simulink model "steering_pad_test_dual"  (R2024b)
settings: Solver=VariableStepAuto  StartTime=0.0  StopTime=10  FixedStep=0.001  RelTol=1e-4
undefined symbols (not defined in the file or in its folder): car
libraries: slpidlib x2, vehdynlibsteering x1, autolibshared x1
settings Model: Creator=Carlo  LastModifiedBy=Carlo
settings SolverCC: ZeroCrossAlgorithm=Adaptive
settings DebuggingCC: IgnoredZcDiagnostic=none

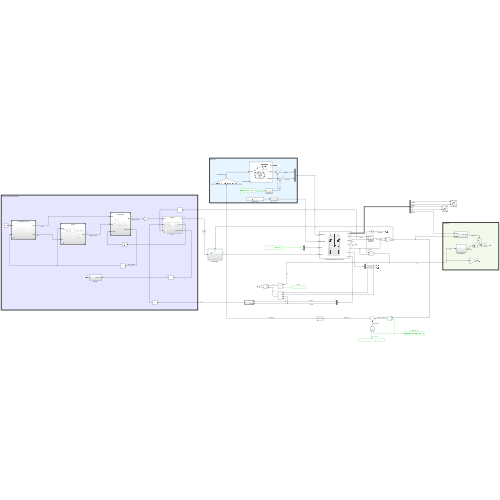
[thumbnail: Simulink's stored preview of the top-level diagram]
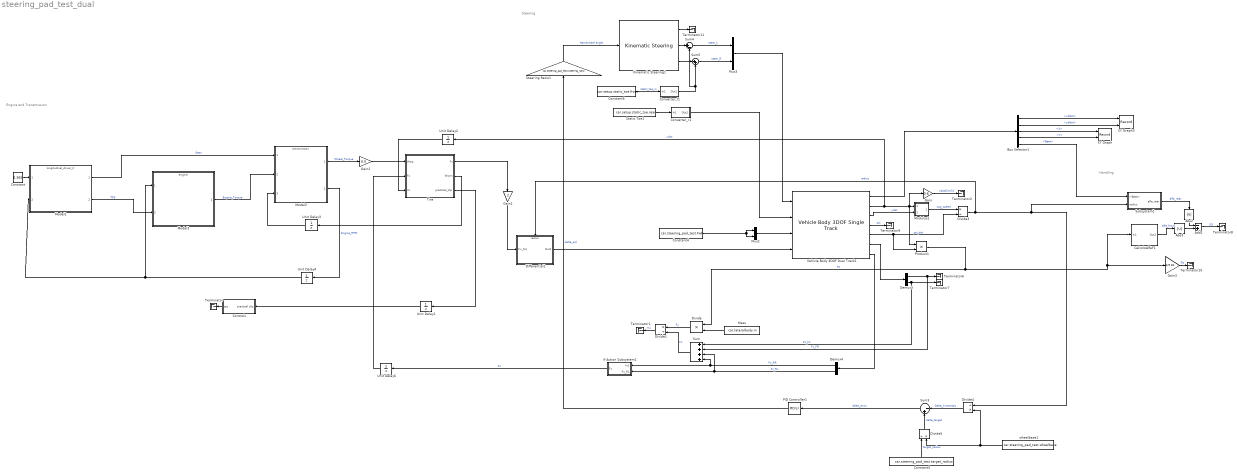
== system steering_pad_test_dual ==
  note: Handling
  note: Steering
  note: Engine and Transmission
  Abs2 : Abs  SaturateOnIntegerOverflow=off
  Abs3 : Abs  SaturateOnIntegerOverflow=off
  Add1 : Sum  Inputs=-+
  Bus Selector1 : BusSelector  OutputSignals=BdyFrm.Cg.Acc.xddot,BdyFrm.Cg.Acc.yddot,InertFrm.Cg.Disp.X,InertFrm.Cg.Disp.Y,BdyFrm.Geom.Ang.Beta
  CalcoloAlfaF1 : Subsystem
  Constant : Constant  Value=0.365
  Constant4 : Constant  Value=car.steering_pad_test.FwF
  Constant5 : Constant  Value=car.steering_pad_test.target_radius
  Constant6 : Constant  Value=car.setup.static_toe.front
  Controls : Subsystem
  Converter_f1 : Subsystem
  Converter_r1 : Subsystem
  Demux3 : Demux  Outputs=2
  Demux4 : Demux  Outputs=2
  Differential1 : Subsystem
      settings: PortSchema="{\"entries\":[{\"content\":{\"sides\":[{\"content\":{\"connectorIds\":[\"In1\"]},\"type\":\"ConnectorPlacement.EquallySpacedRectSide\",\"uuid\":\"e0135ed7-8abf-48dc-a26a-f2473ebc5583\"},{\"content\":{\"connectorIds\":[\"Out1\"],\"side\":\"RIGHT\"},\"type\":\"ConnectorPlacement.EquallySpacedRectSide\",\"uuid\":\"62eb6c38-b859-47c0-94be-9d58d81aad83\"},{\"content\":{\"connectorIds\":[\"In2\"],\"side\":\"TOP\"},\"type\":\"ConnectorPlacement.EquallySpacedRectSide\",\"uuid\":\"7d57c051-97d0-4363-afda-d558cd95b86e\"},{\"content\":{\"side\":\"BOTTOM\"},\"type\":\"ConnectorPlacement.EquallySpacedRectSide\",\"uuid\":\"2453ae4c-76f8-40d8-a1dc-17514a77823a\"}]},\"type\":\"ConnectorPlacement.EquallySpacedConnector\",\"uuid\":\"6460a95d-0a38-4080-9ca3-bbd140d34657\"}],\"packageUris\":[\"http://schema.mathworks.com/mf0/Connector/R2020b\"],\"version\":\"1.0\"}"
  Divide : Product  Inputs=**
  Divide1 : Product  Inputs=*/
  Divide3 : Product  Inputs=*/
  Divide4 : Product  Inputs=/*
  Divide5 : Product  Inputs=/*
  Gain : Gain  Gain=3.6
  Gain1 : Gain  Gain=2
  Gain2 : Gain  Gain=0.5
  Gain3 : Gain  Gain=1/9.81
  If Action Subsystem1 : Subsystem  TreatAsAtomicUnit=on
  Kinematic Steering1 : vehdynlibsteering/Kinematic Steering  StrgType=Ackerman  StrgRatioType=Constant  Loc=Front  NrmlFctr=car.kinematic_steering.NrmlFctr  TrckWdth=car.kinematic_steering.TrckWdth  WhlBase=car.kinematic_steering.WhlBase  Db=car.kinematic_steering.Db  StrgRng=car.kinematic_steering.StrgRng  StrgAngBpts="[-6.2832   -5.0265   -3.7699   -2.5133   -1.2566         0    1.2566    2.5133    3.7699    5.0265    6.2832]"  StrgRatioTbl=|  StrgRatio=car.kinematic_steering.StrgRatio  PctAckIn=off  PctAck=car.kinematic_steering.PctAck  PctAckTbl=ones(1,11)*100  StrgArmLngth=0.1  RckCsLngth=0.5  TieRodLngth=0.248  D=0.2  PnnRadius=0.00085818  PnnRadiusTbl="[0.0055    0.0055    0.0056    0.0057    0.0058    0.0057    0.0057    0.0057    0.0056    0.0055    0.0055]"  RodLngth=0.1  ParaArmLngth=0.9  aMode=2
      | [13.5000   13.3750   13.2500   13.1250   13.0000   13.0000   13.0000   13.1250   13.2500   13.3750   13.5000
      | ]
  Mass : Constant  Value=car.lateralbody.m
  Model1 : ModelReference  ModelNameDialog=longitudinal_driver_2.slx  SimulationMode=Normal  ModelReferenceVersion=1.7
  Model2 : ModelReference  ModelNameDialog=transmission.slx  SimulationMode=Normal  ModelReferenceVersion=1.12
  Model3 : ModelReference  ModelNameDialog=engine.slx  SimulationMode=Normal  ModelReferenceVersion=1.18
  Modulus1 : Subsystem
  Mux2 : Mux  Inputs=2
  Mux3 : Mux  Inputs=2
  PID Controller1 : slpidlib/PID Controller  Controller=PID  Form=Parallel  TimeDomain=Continuous-time  UseExternalTs=off  SampleTime=-1  IntegratorMethod=Forward Euler  FilterMethod=Forward Euler  ControllerParametersSource=internal  P=car.steering_pad_test.PID.P  I=car.steering_pad_test.PID.I  UseKiTs=off  D=car.steering_pad_test.PID.D  UseExternalDerivativeSource=off  N=car.steering_pad_test.PID.N  UseFilter=on  TunerSelectOption=Transfer Function Based (PID Tuner App)  InitialConditionSource=internal  InitialConditionForIntegrator=0  InitialConditionForFilter=0  DifferentiatorICPrevScaledInput=0  ExternalReset=none  TrackingMode=off  Kt=1  LimitOutput=off  SatLimitsSource=internal  UpperSaturationLimit=inf  LowerSaturationLimit=-inf  LinearizeAsGain=on  AntiWindupMode=none  Kb=1  LimitIntegrator=off  UpperIntegratorSaturationLimit=inf  LowerIntegratorSaturationLimit=-inf  POutMin=[]  POutMax=[]  IOutMin=[]  IOutMax=[]  DOutMin=[]  DOutMax=[]  NOutMin=[]  NOutMax=[]  SumOutMin=[]  SumOutMax=[]  SaturationOutMin=[]  SaturationOutMax=[]  PParamMin=[]  PParamMax=[]  IParamMin=[]  IParamMax=[]  DParamMin=[]  DParamMax=[]  NParamMin=[]  NParamMax=[]  KbParamMin=[]  KbParamMax=[]  KtParamMin=[]  KtParamMax=[]  KbOutMin=[]  KbOutMax=[]  KtOutMin=[]  KtOutMax=[]  IntegratorOutMin=[]  IntegratorOutMax=[]  FilterOutMin=[]  FilterOutMax=[]  SumI1OutMin=[]  SumI1OutMax=[]  SumI2OutMin=[]  SumI2OutMax=[]  SumI3OutMin=[]  SumI3OutMax=[]  SumI4OutMin=[]  SumI4OutMax=[]  SumDOutMin=[]  SumDOutMax=[]  DifferentiatorOutMin=[]  DifferentiatorOutMax=[]  FilterDiffOutCoefMin=[]  FilterDiffOutCoefMax=[]  ReciprocalOutMin=[]  ReciprocalOutMax=[]  SumDenOutMin=[]  SumDenOutMax=[]  SumNumOutMin=[]  SumNumOutMax=[]  DivideOutMin=[]  DivideOutMax=[]  UdiffTsProdOutMin=[]  UdiffTsProdOutMax=[]  NTsProdOutMin=[]  NTsProdOutMax=[]  UintegralTsProdOutMin=[]  UintegralTsProdOutMax=[]  UngainTsProdOutMin=[]  UngainTsProdOutMax=[]  ClampingZeroOutDataTypeStr=Inherit: Inherit via back propagation  ClampingZeroOutMin=[]  ClampingZeroOutMax=[]  FilterDenConstantOutDataTypeStr=Inherit: Inherit via back propagation  FilterDenConstantOutMin=[]  FilterDenConstantOutMax=[]  PCopyOutDataTypeStr=Inherit: Inherit via back propagation  PCopyOutMin=[]  PCopyOutMax=[]  NCopyOutDataTypeStr=Inherit: Inherit via back propagation  NCopyOutMin=[]  NCopyOutMax=[]  IntegratorContinuousStateAttributes=''  IntegratorStateMustResolveToSignalObject=off  IntegratorRTWStateStorageClass=Auto  FilterContinuousStateAttributes=''  FilterStateMustResolveToSignalObject=off  FilterRTWStateStorageClass=Auto  ParallelPVariant=InternalParameters  IdealPVariant=Disabled  IVariant=InternalParameters  DVariant=InternalParameters  IntegratorVariant=Continuous  SatVariant=Disabled  AWVariant=Passthrough  PCopyVariant=Disabled  TRVariant=Disabled  FdbkBlocksVariant=Forward  IdealPFdbkVariant=Disabled  SatFdbkVariant=Disabled  DerivativeFilterVariant=ContFilter  NVariant=InternalParameters  NCopyVariant=Disabled  FilterICVariant=InternalICsFilter  IntegratorICVariant=InternalICs  ExternalResetVariant=Disabled  TRSumVariant=Passthrough  SumFdbkVariant=Disabled  SumVariant=Sum_PID  TsampFilterVariant=InternalTs  TsampNgainVariant=Passthrough  TsampIntegralVariant=Disabled_SignalSpec  ExternalSaturationOutDataTypeStr=Inherit: Same as second input  DerivativeSourceVariant=ErrorSignal  PreIntVariant=InternalPreInt
  Product1 : Product
  Static Toe1 : Constant  Value=car.setup.static_toe.rear
  Steering Ratio1 : Gain  Gain=car.steering_pad_test.steering_ratio
  Subsystem1 : Subsystem
  Sum : Sum  Inputs=++++
  Sum3 : Sum  Inputs=|-+
  Sum4 : Sum  Inputs=|+-
  Sum5 : Sum  Inputs=|++
  Terminator{,1..2,6..11} (9 alike) : Terminator
  Tire : Subsystem  Variant=on
  Unit Delay1 : UnitDelay  SampleTime=-1  HasFrameUpgradeWarning=on
  Unit Delay2 : UnitDelay  InitialCondition=car.initialconditions.xdot  SampleTime=-1  HasFrameUpgradeWarning=on
  Unit Delay3 : UnitDelay  InitialCondition=car.initialconditions.Wrpm  SampleTime=-1  HasFrameUpgradeWarning=on
  Unit Delay4 : UnitDelay  InitialCondition=car.initialconditions.EngineRPM  SampleTime=-1  HasFrameUpgradeWarning=on
  Unit Delay6 : UnitDelay  SampleTime=-1  HasFrameUpgradeWarning=on
  Vehicle Body 3DOF Dual Track1 : autolibshared/Vehicle Body 3DOF Single Track  trackMode=Dual  inputMode=External longitudinal forces  frontSteerMode=on  rearSteerMode=on  windMode=off  muMode=off  extFMode=off  extMMode=off  htchFMode=off  htchMMode=off  extXo=off  extpsio=off  extxdoto=off  extro=off  extYo=off  extTamb=off  extydoto=off  aMode=2  NF=car.lateralbody.NF  NR=car.lateralbody.NR  m=car.lateralbody.m  a=car.lateralbody.a  b=car.lateralbody.b  h=car.lateralbody.h  dh=1  hh=0.2  X_o=car.lateralbody.X_o  xdot_o=car.lateralbody.xdot_o  CalphaMode=off  sigmaMode=on  d=car.lateralbody.d  hl=0  w=car.lateral.body.w  Cy_f=car.lateralbody.Cy_f  Cy_r=car.lateralbody.Cy_r  sigma_f=car.lateralbody.sigma_f  sigma_r=car.lateralbody.sigma_r  alpha_f_brk=[-.1 .1]  Cy_f_data=[-9e3 9e3]  alpha_r_brk=[-.1 .1]  Cy_r_data=[-9e3 9e3]  Y_o=car.lateralbody.Y_o  ydot_o=car.lateralbody.ydot_o  Izz=car.lateralbody.Izz  psi_o=car.lateralbody.psi_o  r_o=car.lateralbody.r_o  Af=car.lateralbody.Af  Cd=car.lateralbody.Cd  Cl=car.lateralbody.Cl  Cpm=car.lateralbody.Cpm  beta_w=car.lateralbody.beta_w  Cs=car.lateralbody.Cs  Cym=car.lateralbody.Cym  Pabs=car.lateralbody.Pabs  Tair=car.lateralbody.Tair  g=car.lateralbody.g  mu=car.lateralbody.mu  xdot_tol=car.lateralbody.xdot_tol  Fznom=car.lateralbody.Fznom  Fxtire_sat=7e4  Fytire_sat=7e4  longOff=car.lateralbody.longOff  latOff=car.lateralbody.latOff  vertOff=car.lateralbody.vertOff  wrapAng=off
      settings: LibrarySourceBlock=vehdynlibeom/Vehicle Body 3DOF Dual Track
  XY Graph : Record  FileSettingsInternal="{\"entries\":[{\"content\":{\"excelSettings\":{\"content\":{},\"type\":\"Streamout.ExcelSettings\"}},\"type\":\"Streamout.FileSettingStorage\",\"uuid\":\"\"}],\"packageUris\":[\"http:\\/\\/schema.mathworks.com\\/mf0\\/streamout_blocks\\/R2020a\"],\"version\":\"1.0\"}"  Layout=[1 1]  SignalsInternal="{\"entries\":[{\"content\":{\"signals\":[{\"content\":{\"blockPath\":[],\"dimensions\":[1],\"domain\":\"\",\"lineColor\":\"#a2142f\",\"plots\":[ 1 ],\"port\":1,\"sid\":[\"\"],\"signalID\":1,\"signalName\":\"<X>\"},\"type\":\"RecordBlkView.Signal\",\"uuid\":\"\"},{\"content\":{\"blockPath\":[],\"dimensions\":[1],\"domain\":\"\",\"lineColor\":\"#139fff\",\"plots\":[ 1 ],\"port\":2,\"sid\":[\"\"],\"signalID\":2,\"signalName\":\"<Y>\"},\"type\":\"RecordBlkView.Signal\",\"uuid\":\"\"}]},\"type\":\"RecordBlkView.InputSignals\",\"uuid\":\"\"}],\"packageUris\":[\"http:\\/\\/schema.mathworks.com\\/mf0\\/streamout_blocks\\/R2020a\"],\"version\":\"1.0\"}"  VisualizationBindings="{\"xyplotplugin\":{\"info\":[{\"series\":[{\"bindingParametersList\":[{\"parameter\":\"X-Axis\",\"signalID\":1,\"signalName\":\"<X>\"},{\"parameter\":\"Y-Axis\",\"signalID\":2,\"signalName\":\"<Y>\"}],\"seriesID\":0}],\"subplotID\":1}]}}"  CompatibilityTag=XY
  XY Graph3 : Record  FileSettingsInternal="{\"entries\":[{\"content\":{\"excelSettings\":{\"content\":{},\"type\":\"Streamout.ExcelSettings\"}},\"type\":\"Streamout.FileSettingStorage\",\"uuid\":\"\"}],\"packageUris\":[\"http:\\/\\/schema.mathworks.com\\/mf0\\/streamout_blocks\\/R2020a\"],\"version\":\"1.0\"}"  Layout=[1 1]  SignalsInternal="{\"entries\":[{\"content\":{\"signals\":[{\"content\":{\"blockPath\":[],\"dimensions\":[1],\"domain\":\"\",\"lineColor\":\"#fe330a\",\"lineWidth\":2,\"port\":1,\"sid\":[\"\"],\"signalID\":1,\"signalName\":\"<xddot>\"},\"type\":\"RecordBlkView.Signal\",\"uuid\":\"\"},{\"content\":{\"blockPath\":[],\"dimensions\":[1],\"domain\":\"\",\"lineColor\":\"#22b573\",\"lineWidth\":2,\"port\":2,\"sid\":[\"\"],\"signalID\":2,\"signalName\":\"<yddot>\"},\"type\":\"RecordBlkView.Signal\",\"uuid\":\"\"}]},\"type\":\"RecordBlkView.InputSignals\",\"uuid\":\"\"}],\"packageUris\":[\"http:\\/\\/schema.mathworks.com\\/mf0\\/streamout_blocks\\/R2020a\"],\"version\":\"1.0\"}"  VisualizationBindings="{\"xyplotplugin\":{\"info\":[{\"series\":[],\"subplotID\":1}]}}"  CompatibilityTag=XY
  wheelbase1 : Constant  Value=car.steering_pad_test.wheelbase
  wires:
  Unit Delay3/1 -> Model2/3
  Model1/2 -> Model3/2  "TPS"
  Unit Delay4/1 -> Model3/1, Model1/2
  Unit Delay1/1 -> Controls/1(practical slip)
  Tire/3(practical_slip) -> Unit Delay1/1
  Model3/1 -> Model2/2  "Engine_Torque"
  Unit Delay2/1 -> Tire/3(Vx)
  Model1/1 -> Model2/1  "Gear"
  Tire/2(Wrpm) -> Unit Delay3/1
  Model2/1 -> Gain2/1  "Wheel_Torque"
  Model2/2 -> Unit Delay4/1  "Engine_RPM"
  Gain2/1 -> Tire/1(Wtrq)
  Sum3/1 -> PID Controller1/1  "delta_error"
  Bus Selector1/1 -> XY Graph3/1  "<xddot>"
  Modulus1/1(Out1) -> Divide3/1  "cog_speed"
  Bus Selector1/4 -> XY Graph/2  "<Y>"
  PID Controller1/1 -> Steering Ratio1/1  "delta_pid"
  Vehicle Body 3DOF Dual Track1/6 -> Demux3/1
  Bus Selector1/5 -> Subsystem1/1(<Beta>)  "<Beta>"
  Kinematic Steering1/1 -> Terminator11/1
  Bus Selector1/2 -> XY Graph3/2  "<yddot>"
  Divide5/1 -> Sum3/2  "delta_target"
  CalcoloAlfaF1/1(Out1) -> Abs3/1  "alfa_front"
  Constant4/1 -> Mux2/2, Mux2/1
  Constant5/1 -> Divide5/1  "target_radius"
  Subsystem1/1(alfa_rear) -> Abs2/1  "alfa_rear"
  Divide4/1 -> Sum3/1  "Delta_kinematic"
  Mux3/1 -> Vehicle Body 3DOF Dual Track1/1
  Vehicle Body 3DOF Dual Track1/1 -> Bus Selector1/1
  Abs3/1 -> Add1/2
  Sum5/1 -> Mux3/2  "steer_R"
  Kinematic Steering1/3 -> Sum5/1
  Divide3/1 -> Subsystem1/2(radius), Divide4/1, Differential1/2(radius)  "radius"
  Vehicle Body 3DOF Dual Track1/4 -> Terminator9/1  "psi"
  Mux2/1 -> Vehicle Body 3DOF Dual Track1/3
  Vehicle Body 3DOF Dual Track1/2 -> Unit Delay2/1, Gain/1, Modulus1/1(<xdot>), Product1/1  "xdot"
  Differential1/1(Out1) -> Vehicle Body 3DOF Dual Track1/4
  Add1/1 -> Terminator8/1  "US"
  Demux3/1 -> Sum/2, Terminator6/1  "Fz_FR"
  wheelbase1/1 -> Divide4/2, Divide5/2
  Demux3/2 -> Sum/1, Terminator7/1  "Fz_FL"
  Sum4/1 -> Mux3/1  "steer_L"
  Converter_f1/1(Out1) -> Sum4/2, Sum5/2
  Vehicle Body 3DOF Dual Track1/5 -> Product1/2, Divide3/2  "psi_dot"
  Static Toe1/1 -> Converter_r1/1(In1)
  Constant6/1 -> Converter_f1/1(In1)  "static_toe_in"
  Bus Selector1/3 -> XY Graph/1  "<X>"
  Converter_r1/1(Out1) -> Vehicle Body 3DOF Dual Track1/2
  Product1/1 -> Divide/1, CalcoloAlfaF1/1(In1), Gain3/1  "ay"
  Vehicle Body 3DOF Dual Track1/3 -> Modulus1/2(<ydot>)  "ydot"
  Gain3/1 -> Terminator10/1  "Gy"
  Abs2/1 -> Add1/1
  Steering Ratio1/1 -> Kinematic Steering1/1  "Handwheel angle"
  Kinematic Steering1/2 -> Sum4/1
  Demux4/1 -> Sum/4, If Action Subsystem1/1(In1)  "Fz_RR"
  Vehicle Body 3DOF Dual Track1/7 -> Demux4/1
  Demux4/2 -> Sum/3, If Action Subsystem1/2(Fz_RL)  "Fz_RL"
  If Action Subsystem1/1(Fz) -> Unit Delay6/1  "Fz"
  Unit Delay6/1 -> Tire/2(Fz)
  Constant/1 -> Model1/1
  Tire/1(Fx) -> Gain1/1
  Gain1/1 -> Differential1/1(Fx_tot)
  Controls/1(tps) -> Terminator/1
  Mass/1 -> Divide/2
  Divide/1 -> Divide1/1  "Fy"
  Divide1/1 -> Terminator1/1  "mu"
  Gain/1 -> Terminator2/1  "xdot[km/h]"
  Sum/1 -> Divide1/2  "Fz"

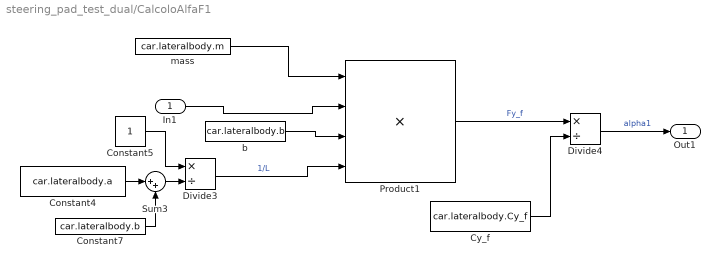
== system steering_pad_test_dual/CalcoloAlfaF1 ==
  In1 : Inport
  Constant4 : Constant  Value=car.lateralbody.a
  Constant5 : Constant
  Constant7 : Constant  Value=car.lateralbody.b
  Cy_f : Constant  Value=car.lateralbody.Cy_f
  Divide3 : Product  Inputs=*/
  Divide4 : Product  Inputs=*/
  Product1 : Product  Inputs=4
  Sum3 : Sum  Inputs=|++
  b : Constant  Value=car.lateralbody.b
  mass : Constant  Value=car.lateralbody.m
  Out1 : Outport
  wires:
  mass/1 -> Product1/1
  Divide3/1 -> Product1/4  "1/L"
  Sum3/1 -> Divide3/2
  b/1 -> Product1/3
  Constant4/1 -> Sum3/1
  Constant5/1 -> Divide3/1
  Divide4/1 -> Out1/1  "alpha1"
  Constant7/1 -> Sum3/2
  Product1/1 -> Divide4/1  "Fy_f"
  Cy_f/1 -> Divide4/2
  In1/1 -> Product1/2

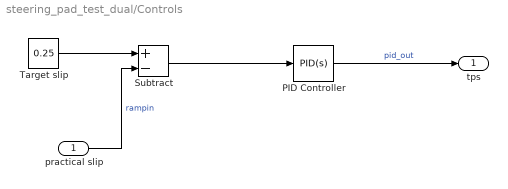
== system steering_pad_test_dual/Controls ==
  practical slip : Inport
  PID Controller : slpidlib/PID Controller  Controller=PID  Form=Parallel  TimeDomain=Continuous-time  UseExternalTs=off  SampleTime=-1  IntegratorMethod=Forward Euler  FilterMethod=Forward Euler  ControllerParametersSource=internal  P=7.5  I=0.75  UseKiTs=off  D=0.075  UseExternalDerivativeSource=off  N=0  UseFilter=on  TunerSelectOption=Transfer Function Based (PID Tuner App)  InitialConditionSource=internal  InitialConditionForIntegrator=0  InitialConditionForFilter=0  DifferentiatorICPrevScaledInput=0  ExternalReset=none  TrackingMode=off  Kt=1  LimitOutput=on  SatLimitsSource=internal  UpperSaturationLimit=1  LowerSaturationLimit=0  LinearizeAsGain=on  AntiWindupMode=none  Kb=1  LimitIntegrator=off  UpperIntegratorSaturationLimit=inf  LowerIntegratorSaturationLimit=-inf  POutMin=[]  POutMax=[]  IOutMin=[]  IOutMax=[]  DOutMin=[]  DOutMax=[]  NOutMin=[]  NOutMax=[]  SumOutMin=[]  SumOutMax=[]  SaturationOutMin=[]  SaturationOutMax=[]  PParamMin=[]  PParamMax=[]  IParamMin=[]  IParamMax=[]  DParamMin=[]  DParamMax=[]  NParamMin=[]  NParamMax=[]  KbParamMin=[]  KbParamMax=[]  KtParamMin=[]  KtParamMax=[]  KbOutMin=[]  KbOutMax=[]  KtOutMin=[]  KtOutMax=[]  IntegratorOutMin=[]  IntegratorOutMax=[]  FilterOutMin=[]  FilterOutMax=[]  SumI1OutMin=[]  SumI1OutMax=[]  SumI2OutMin=[]  SumI2OutMax=[]  SumI3OutMin=[]  SumI3OutMax=[]  SumI4OutMin=[]  SumI4OutMax=[]  SumDOutMin=[]  SumDOutMax=[]  DifferentiatorOutMin=[]  DifferentiatorOutMax=[]  FilterDiffOutCoefMin=[]  FilterDiffOutCoefMax=[]  ReciprocalOutMin=[]  ReciprocalOutMax=[]  SumDenOutMin=[]  SumDenOutMax=[]  SumNumOutMin=[]  SumNumOutMax=[]  DivideOutMin=[]  DivideOutMax=[]  UdiffTsProdOutMin=[]  UdiffTsProdOutMax=[]  NTsProdOutMin=[]  NTsProdOutMax=[]  UintegralTsProdOutMin=[]  UintegralTsProdOutMax=[]  UngainTsProdOutMin=[]  UngainTsProdOutMax=[]  ClampingZeroOutDataTypeStr=Inherit: Inherit via back propagation  ClampingZeroOutMin=[]  ClampingZeroOutMax=[]  FilterDenConstantOutDataTypeStr=Inherit: Inherit via back propagation  FilterDenConstantOutMin=[]  FilterDenConstantOutMax=[]  PCopyOutDataTypeStr=Inherit: Inherit via back propagation  PCopyOutMin=[]  PCopyOutMax=[]  NCopyOutDataTypeStr=Inherit: Inherit via back propagation  NCopyOutMin=[]  NCopyOutMax=[]  IntegratorContinuousStateAttributes=''  IntegratorStateMustResolveToSignalObject=off  IntegratorRTWStateStorageClass=Auto  FilterContinuousStateAttributes=''  FilterStateMustResolveToSignalObject=off  FilterRTWStateStorageClass=Auto  ParallelPVariant=InternalParameters  IdealPVariant=Disabled  IVariant=InternalParameters  DVariant=InternalParameters  IntegratorVariant=Continuous  SatVariant=Enabled  AWVariant=Passthrough  PCopyVariant=Disabled  TRVariant=Disabled  FdbkBlocksVariant=Forward  IdealPFdbkVariant=Disabled  SatFdbkVariant=Disabled  DerivativeFilterVariant=ContFilter  NVariant=InternalParameters  NCopyVariant=Disabled  FilterICVariant=InternalICsFilter  IntegratorICVariant=InternalICs  ExternalResetVariant=Disabled  TRSumVariant=Passthrough  SumFdbkVariant=Disabled  SumVariant=Sum_PID  TsampFilterVariant=InternalTs  TsampNgainVariant=Passthrough  TsampIntegralVariant=Disabled_SignalSpec  ExternalSaturationOutDataTypeStr=Inherit: Same as second input  DerivativeSourceVariant=ErrorSignal  PreIntVariant=InternalPreInt
  Subtract : Sum  Inputs=+-
  Target slip : Constant  Value=0.25
  tps : Outport
  wires:
  practical slip/1 -> Subtract/2  "rampin"
  Target slip/1 -> Subtract/1
  Subtract/1 -> PID Controller/1
  PID Controller/1 -> tps/1  "pid_out"

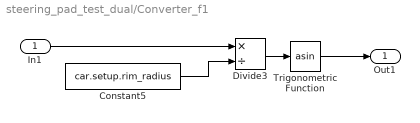
== system steering_pad_test_dual/Converter_f1 ==
  In1 : Inport
  Constant5 : Constant  Value=car.setup.rim_radius  VectorParams1D=off
  Divide3 : Product  Inputs=*/
  Trigonometric Function : Trigonometry  Operator=asin
  Out1 : Outport
  wires:
  In1/1 -> Divide3/1
  Divide3/1 -> Trigonometric Function/1
  Trigonometric Function/1 -> Out1/1
  Constant5/1 -> Divide3/2

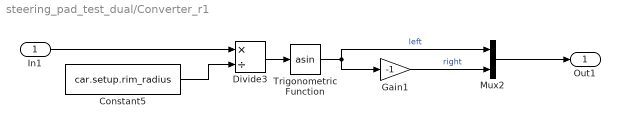
== system steering_pad_test_dual/Converter_r1 ==
  In1 : Inport
  Constant5 : Constant  Value=car.setup.rim_radius  VectorParams1D=off
  Divide3 : Product  Inputs=*/
  Gain1 : Gain  Gain=-1
  Mux2 : Mux  Inputs=2
  Trigonometric Function : Trigonometry  Operator=asin
  Out1 : Outport
  wires:
  In1/1 -> Divide3/1
  Gain1/1 -> Mux2/2  "right"
  Divide3/1 -> Trigonometric Function/1
  Trigonometric Function/1 -> Mux2/1, Gain1/1  "left"
  Constant5/1 -> Divide3/2
  Mux2/1 -> Out1/1

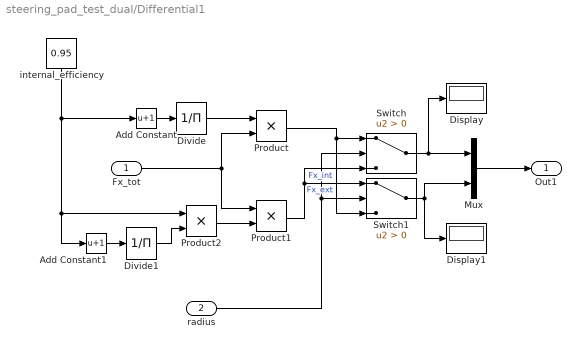
== system steering_pad_test_dual/Differential1 ==
  Fx_tot : Inport
  radius : Inport  Port=2
  Add Constant : Bias  Bias=1  SaturateOnIntegerOverflow=off
  Add Constant1 : Bias  Bias=1  SaturateOnIntegerOverflow=off
  Display : Display
  Display1 : Display
  Divide : Product  Inputs=/
  Divide1 : Product  Inputs=/
  Mux : Mux  Inputs=2
  Product : Product
  Product1 : Product
  Product2 : Product
  Switch : Switch  Criteria=u2 > Threshold  SaturateOnIntegerOverflow=off  InputSameDT=off
  Switch1 : Switch  Criteria=u2 > Threshold  SaturateOnIntegerOverflow=off  InputSameDT=off
  internal_efficiency : Constant  Value=0.95
  Out1 : Outport
  wires:
  Mux/1 -> Out1/1
  Fx_tot/1 -> Product1/1, Product/2
  Add Constant/1 -> Divide/1
  internal_efficiency/1 -> Product2/1, Add Constant1/1, Add Constant/1
  Divide/1 -> Product/1
  Add Constant1/1 -> Divide1/1
  Divide1/1 -> Product2/2
  Product2/1 -> Product1/2
  Product/1 -> Switch/1, Switch1/3  "Fx_int"
  radius/1 -> Switch1/2, Switch/2
  Switch/1 -> Display/1, Mux/1
  Product1/1 -> Switch1/1, Switch/3  "Fx_ext"
  Switch1/1 -> Display1/1, Mux/2

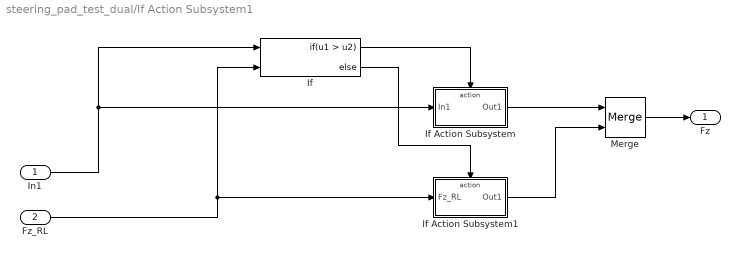
== system steering_pad_test_dual/If Action Subsystem1 ==
  In1 : Inport
  Fz_RL : Inport  Port=2
  If : If  NumInputs=2  IfExpression=u1 > u2
  If Action Subsystem : Subsystem  TreatAsAtomicUnit=on
  If Action Subsystem1 : Subsystem  TreatAsAtomicUnit=on
  Merge : Merge
  Fz : Outport
  wires:
  In1/1 -> If Action Subsystem/1(In1), If/1
  Fz_RL/1 -> If/2, If Action Subsystem1/1(Fz_RL)
  If/1 -> If Action Subsystem/Action
  If Action Subsystem/1(Out1) -> Merge/1
  If/2 -> If Action Subsystem1/Action
  If Action Subsystem1/1(Out1) -> Merge/2
  Merge/1 -> Fz/1

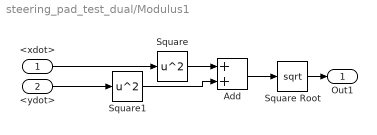
== system steering_pad_test_dual/Modulus1 ==
  <xdot> : Inport
  <ydot> : Inport  Port=2
  Add : Sum
  Square : Math  Operator=square
  Square Root : Sqrt
  Square1 : Math  Operator=square
  Out1 : Outport
  wires:
  Add/1 -> Square Root/1
  Square/1 -> Add/1
  Square1/1 -> Add/2
  Square Root/1 -> Out1/1
  <ydot>/1 -> Square1/1
  <xdot>/1 -> Square/1

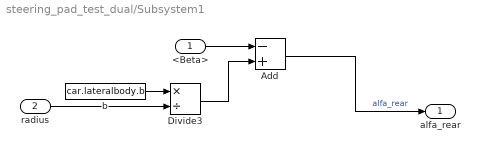
== system steering_pad_test_dual/Subsystem1 ==
  <Beta> : Inport
  radius : Inport  Port=2
  Add : Sum  Inputs=-+
  Divide3 : Product  Inputs=*/
  b : Constant  Value=car.lateralbody.b
  alfa_rear : Outport
  wires:
  radius/1 -> Divide3/2
  Add/1 -> alfa_rear/1  "alfa_rear"
  Divide3/1 -> Add/2
  b/1 -> Divide3/1
  <Beta>/1 -> Add/1

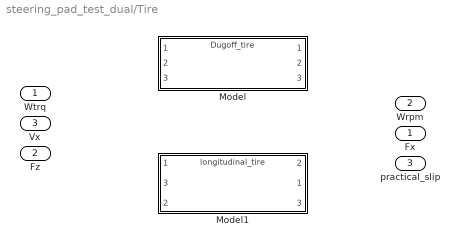
== system steering_pad_test_dual/Tire ==
  Wtrq : Inport
  Fz : Inport  Port=2
  Vx : Inport  Port=3
  Model : ModelReference  DisableCoverage=on  ModelNameDialog=Dugoff_tire.slx  SimulationMode=Normal  VariantControl=false  ModelReferenceVersion=2.16
  Model1 : ModelReference  ModelNameDialog=longitudinal_tire.slx  SimulationMode=Normal  VariantControl=true  ModelReferenceVersion=3.7
      settings: PortSchema="{\"entries\":[{\"content\":{\"sides\":[{\"content\":{\"connectorIds\":[\"In1\",\"In3\",\"In2\"]},\"type\":\"ConnectorPlacement.EquallySpacedRectSide\",\"uuid\":\"5eba1a74-bd07-49e9-ac91-356b950fcd72\"},{\"content\":{\"connectorIds\":[\"Out2\",\"Out1\",\"Out3\"],\"side\":\"RIGHT\"},\"type\":\"ConnectorPlacement.EquallySpacedRectSide\",\"uuid\":\"1040ce78-c535-419a-aa8f-ad6fbf19e979\"},{\"content\":{\"side\":\"TOP\"},\"type\":\"ConnectorPlacement.EquallySpacedRectSide\",\"uuid\":\"ba0f3e1f-76c3-4461-91cd-c7f47b575855\"}]},\"type\":\"ConnectorPlacement.EquallySpacedConnector\",\"uuid\":\"77c71335-a5e7-4e66-a78b-88921c7c7d22\"}],\"packageUris\":[\"http://schema.mathworks.com/mf0/Connector/R2020b\"],\"version\":\"1.0\"}"
  Fx : Outport
  Wrpm : Outport  Port=2
  practical_slip : Outport  Port=3

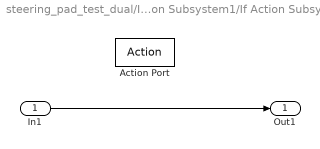
== system steering_pad_test_dual/If Action Subsystem1/If Action Subsystem ==
  In1 : Inport
  Action Port : ActionPort  ActionPortLabel=if(u1 > u2)
  Out1 : Outport
  wires:
  In1/1 -> Out1/1

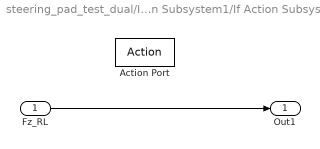
== system steering_pad_test_dual/If Action Subsystem1/If Action Subsystem1 ==
  Fz_RL : Inport
  Action Port : ActionPort  ActionPortLabel=else
  Out1 : Outport
  wires:
  Fz_RL/1 -> Out1/1
